simulink model "ES229A_HwTqCorrln"  (R2013b)
settings: Solver=FixedStepDiscrete  SolverMode=SingleTasking  StartTime=0.0  StopTime=1  FixedStep=0.002  RelTol=1e-3
undefined symbols (not defined in the file): ARCHGLBPRM_100MILLISEC_SEC_F32, FLTINJ_HWTQCORRLN_HWTQIDPTSIG, HwTqCorrlnChACmnModCmpLpFilActvnThd, HwTqCorrlnChACmnModCmpLpFilOutpLim, HwTqCorrlnChAImdtCorrlnChkFailThd, HwTqCorrlnChAImdtCorrlnChkPassThd, HwTqCorrlnChAStabStClrFltThd, HwTqCorrlnChAStabStSetFltThd, HwTqCorrlnChATqSumMaxLim, HwTqCorrlnChATraSumClrFltThd, HwTqCorrlnChATraSumSetFltThd, HwTqCorrlnChBCmnModCmpLpFilActvnThd, HwTqCorrlnChBCmnModCmpLpFilOutpLim, HwTqCorrlnChBImdtCorrlnChkFailThd, HwTqCorrlnChBImdtCorrlnChkPassThd, HwTqCorrlnChBStabStClrFltThd, HwTqCorrlnChBStabStSetFltThd, HwTqCorrlnChBTqSumMaxLim, HwTqCorrlnChBTraSumClrFltThd, HwTqCorrlnChBTraSumSetFltThd, HwTqCorrlnMaxStallTqA, HwTqCorrlnMaxStallTqB, HwTqCorrlnMaxStallTqC, HwTqCorrlnMaxStallTqD, HWTQSCA_CNT_U08, NtcNr1, NtcSts1, PARAMETERBYTE_CNT_U08, sigbuilder_block, SigQlfr1, STABSTLPFILSTVARIDELTALIM_HWNWTMTR_F32
libraries: simulink x25, Fil x12, NxtrLim x10, NxtrAbslt x6, FixdToFloat x2, FloatToFixdWithRound x2, LnrIntrpn x2, NxtrNvM x2
(part 3 of 4)

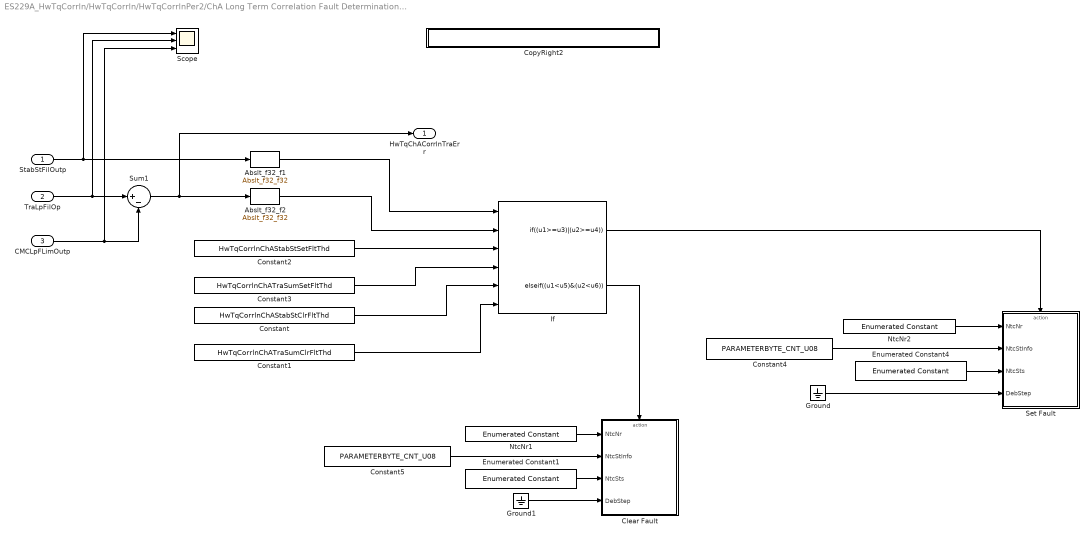
== system ES229A_HwTqCorrln/HwTqCorrln/HwTqCorrlnPer2/ChA Long Term Correlation Fault Determination/Ch A Set//Clear Fault ==
  StabStFilOutp : Inport
  TraLpFilOp : Inport  Port=2
  CMCLpFLimOutp : Inport  Port=3
  Abslt_f32_f1 : NxtrAbslt/Abslt_f32_f32  SFunctionSpec=single y1 = Abslt_f32_f32(single u1)
      settings: AttributesFormatString=%<Name>
  Abslt_f32_f2 : NxtrAbslt/Abslt_f32_f32  SFunctionSpec=single y1 = Abslt_f32_f32(single u1)
      settings: AttributesFormatString=%<Name>
  Clear Fault : Subsystem  mask(SetNTC){}
      mask help: SetNTC library block
  Constant : Constant  Value=HwTqCorrlnChAStabStClrFltThd
  Constant1 : Constant  Value=HwTqCorrlnChATraSumClrFltThd
  Constant2 : Constant  Value=HwTqCorrlnChAStabStSetFltThd
  Constant3 : Constant  Value=HwTqCorrlnChATraSumSetFltThd
  Constant4 : Constant  Value=PARAMETERBYTE_CNT_U08
  Constant5 : Constant  Value=PARAMETERBYTE_CNT_U08
  CopyRight2 : Subsystem  Description=|  mask(Copyright Information){none=on}
      | Copyright info block.                                               
      |                                                                     
      | Place copyright information at the top of every subsystem in design.
      mask prompts: none "No parameters"
      mask help: Place copyright information at the top of every subsystem in design.
      mask Display:
      | NxtrConf = 'Nexteer Confidential';
      | 
      | sys = bdroot; %handle for the current model ("system")
      | first = get_param(sys,'Created');
      | first = first(end-3:end);  %year is last four digits
      | 
      | last = get_param(sys,'LastModifiedDate');
      | if isempty(last)
      |     last = datestr(now,'yyyy');
      | else
      |     last = last(end-3:end);
      | end
      | 
      | if strcmp(first,last)
      |     fprintf('%s -- Copyright %s Nexteer',NxtrConf,first)
      | else
      |     fprintf('%s -- %s%s- %s Nexteer',NxtrConf,char(169),first,last)
      | end
  Enumerated Constant1 : simulink/Sources/Enumerated Constant  OutDataTypeStr=Enum: NtcSts1  Value=NtcSts1.NTCSTS_PASSD  SampleTime=inf
  Enumerated Constant4 : simulink/Sources/Enumerated Constant  OutDataTypeStr=Enum: NtcSts1  Value=NtcSts1.NTCSTS_FAILD  SampleTime=inf
  Ground : Ground
  Ground1 : Ground
  If : If  NumInputs=6  IfExpression=(u1>=u3)|(u2>=u4)  ElseIfExpressions=(u1<u5)&(u2<u6)  ShowElse=off
  NtcNr1 : simulink/Sources/Enumerated Constant  OutDataTypeStr=Enum: NtcNr1  Value=NtcNr1.NTCNR_0X070  SampleTime=inf
  NtcNr2 : simulink/Sources/Enumerated Constant  OutDataTypeStr=Enum: NtcNr1  Value=NtcNr1.NTCNR_0X070  SampleTime=inf
  Scope : Scope  NumInputPorts=3
      settings: TimeRange=auto  LimitDataPoints=on  MaxDataPoints=5000  SaveToWorkspace=off  SaveName=ScopeData3  YMin=-5~-5~-5  YMax=5~5~5  SampleTime=-1
  Set Fault : Subsystem  mask(SetNTC){}
      mask help: SetNTC library block
  Sum1 : Sum  RequirementInfo={} %GIDa_36dd93a3_b811_40f0_b925_6a2a9cd5f46c  Inputs=|+-
  HwTqChACorrlnTraErr : Outport
  wires:
  Abslt_f32_f1/1 -> If/1
  Constant/1 -> If/5
  Constant1/1 -> If/6
  If/1 -> Set Fault/Action
  NtcNr2/1 -> Set Fault/1(NtcNr)
  Constant4/1 -> Set Fault/2(NtcStInfo)
  Enumerated Constant4/1 -> Set Fault/3(NtcSts)
  Ground/1 -> Set Fault/4(DebStep)
  Constant3/1 -> If/4
  If/2 -> Clear Fault/Action
  NtcNr1/1 -> Clear Fault/1(NtcNr)
  Constant5/1 -> Clear Fault/2(NtcStInfo)
  Enumerated Constant1/1 -> Clear Fault/3(NtcSts)
  Ground1/1 -> Clear Fault/4(DebStep)
  StabStFilOutp/1 -> Scope/1, Abslt_f32_f1/1
  Sum1/1 -> HwTqChACorrlnTraErr/1, Abslt_f32_f2/1
  Abslt_f32_f2/1 -> If/2
  Constant2/1 -> If/3
  CMCLpFLimOutp/1 -> Scope/3, Sum1/2
  TraLpFilOp/1 -> Scope/2, Sum1/1

== system ES229A_HwTqCorrln/HwTqCorrln/HwTqCorrlnPer2/ChA Long Term Correlation Fault Determination/Ch A Variable Fc Transient Fault LPF ==
  note: Add data type conversion Inp and out of table
  TrqSumLmt : Inport
  Abslt_f32_f32 : NxtrAbslt/Abslt_f32_f32  SFunctionSpec=single y1 = Abslt_f32_f32(single u1)
      settings: AttributesFormatString=%<Name>
  CopyRight2 : Subsystem  Description=|  mask(Copyright Information){none=on}
      | Copyright info block.                                               
      |                                                                     
      | Place copyright information at the top of every subsystem in design.
      mask prompts: none "No parameters"
      mask help: Place copyright information at the top of every subsystem in design.
      mask Display:
      | NxtrConf = 'Nexteer Confidential';
      | 
      | sys = bdroot; %handle for the current model ("system")
      | first = get_param(sys,'Created');
      | first = first(end-3:end);  %year is last four digits
      | 
      | last = get_param(sys,'LastModifiedDate');
      | if isempty(last)
      |     last = datestr(now,'yyyy');
      | else
      |     last = last(end-3:end);
      | end
      | 
      | if strcmp(first,last)
      |     fprintf('%s -- Copyright %s Nexteer',NxtrConf,first)
      | else
      |     fprintf('%s -- %s%s- %s Nexteer',NxtrConf,char(169),first,last)
      | end
  FilLpUpdGain : Fil/FilLpUpdGain  Priority=2  Ts=single(0.004)  StVar=HwTqChATraLpFil
      settings: AttributesFormatString=|
      | Ts: %<Ts>
      | StVar: %<StVar>
      | Priority: %<Priority>
  FilLpUpdOutp : Fil/FilLpUpdOutp  Priority=3  StVar=HwTqChATraLpFil
      settings: AttributesFormatString=|
      | StVar: %<StVar>
      | Priority: %<Priority>
  FixdToFloat_f32_u16 : FixdToFloat/FixdToFloat_f32_u16  Param1=10
  FloatToFixdWithRound_u16_f32 : FloatToFixdWithRound/FloatToFixdWithRound_u16_f32  Param1=11
  LnrIntrpn_u16_u16VariXu16VariY : LnrIntrpn/LnrIntrpn_u16_u16VariXu16VariY  Priority=1  XTbl=HwTqCorrlnChATraLpFilX  YTbl=HwTqCorrlnChATraLpFilY
      settings: AttributesFormatString=|
      | Lnr ( u16VariX , u16VariY )
      | Priority: %<Priority>
  TraLpFilOp : Outport
  wires:
  TrqSumLmt/1 -> Abslt_f32_f32/1, FilLpUpdOutp/1
  Abslt_f32_f32/1 -> FloatToFixdWithRound_u16_f32/1
  LnrIntrpn_u16_u16VariXu16VariY/1 -> FixdToFloat_f32_u16/1
  FloatToFixdWithRound_u16_f32/1 -> LnrIntrpn_u16_u16VariXu16VariY/1
  FixdToFloat_f32_u16/1 -> FilLpUpdGain/1
  FilLpUpdOutp/1 -> TraLpFilOp/1

== system ES229A_HwTqCorrln/HwTqCorrln/HwTqCorrlnPer2/ChA Long Term Correlation Fault Determination/ChA CMC LPF Limit ==
  Constant1 : Constant  RequirementInfo={} %GIDa_72eaf94a_e667_4cbf_a56b_a3f43667705d  Value=-1  OutDataTypeStr=single
  Constant2 : Constant  RequirementInfo={} %GIDa_dca1123b_deb2_4786_b31b_bd2c5c60cbec  Value=HwTqCorrlnChACmnModCmpLpFilOutpLim
  CopyRight2 : Subsystem  Description=|  mask(Copyright Information){none=on}
      | Copyright info block.                                               
      |                                                                     
      | Place copyright information at the top of every subsystem in design.
      mask prompts: none "No parameters"
      mask help: Place copyright information at the top of every subsystem in design.
      mask Display:
      | NxtrConf = 'Nexteer Confidential';
      | 
      | sys = bdroot; %handle for the current model ("system")
      | first = get_param(sys,'Created');
      | first = first(end-3:end);  %year is last four digits
      | 
      | last = get_param(sys,'LastModifiedDate');
      | if isempty(last)
      |     last = datestr(now,'yyyy');
      | else
      |     last = last(end-3:end);
      | end
      | 
      | if strcmp(first,last)
      |     fprintf('%s -- Copyright %s Nexteer',NxtrConf,first)
      | else
      |     fprintf('%s -- %s%s- %s Nexteer',NxtrConf,char(169),first,last)
      | end
  Data Store Read1 : DataStoreRead  DataStoreName=HwTqChACmnModCmpLpFil  DataStoreElements=HwTqChACmnModCmpLpFil.FilSt
  LimDyn_f32 : NxtrLim/LimDyn_f32  RequirementInfo={} %GIDa_1c7be57d_faef_4bd1_a7ab_75ed3e2b2752
  Product : Product  RequirementInfo={} %GIDa_d7a373ed_dd9b_4899_a765_22120a24fae2  OutDataTypeStr=single
  CmnModCmpLpFilOutpLmt : Outport
  wires:
  LimDyn_f32/1 -> CmnModCmpLpFilOutpLmt/1
  Data Store Read1/1 -> LimDyn_f32/1
  Constant2/1 -> Product/2, LimDyn_f32/3
  Constant1/1 -> Product/1
  Product/1 -> LimDyn_f32/2

== system ES229A_HwTqCorrln/HwTqCorrln/HwTqCorrlnPer2/ChA Long Term Correlation Fault Determination/ChA Trq Sum Limit ==
  In1 : Inport
  In2 : Inport  Port=2
  Constant : Constant  Value=HWTQSCA_CNT_U08
  Constant1 : Constant  Value=-1  OutDataTypeStr=single
  Constant3 : Constant  RequirementInfo={} %GIDa_078b91aa_a9cb_4a51_ac3c_bc7f46b72b6a  Value=HwTqCorrlnChATqSumMaxLim
  CopyRight2 : Subsystem  Description=|  mask(Copyright Information){none=on}
      | Copyright info block.                                               
      |                                                                     
      | Place copyright information at the top of every subsystem in design.
      mask prompts: none "No parameters"
      mask help: Place copyright information at the top of every subsystem in design.
      mask Display:
      | NxtrConf = 'Nexteer Confidential';
      | 
      | sys = bdroot; %handle for the current model ("system")
      | first = get_param(sys,'Created');
      | first = first(end-3:end);  %year is last four digits
      | 
      | last = get_param(sys,'LastModifiedDate');
      | if isempty(last)
      |     last = datestr(now,'yyyy');
      | else
      |     last = last(end-3:end);
      | end
      | 
      | if strcmp(first,last)
      |     fprintf('%s -- Copyright %s Nexteer',NxtrConf,first)
      | else
      |     fprintf('%s -- %s%s- %s Nexteer',NxtrConf,char(169),first,last)
      | end
  Divide : Product  Inputs=*/
  LimDyn_f32 : NxtrLim/LimDyn_f32
  Product : Product  OutDataTypeStr=single
  Sum : Sum  Inputs=+|-
  Out1 : Outport
  wires:
  In1/1 -> Sum/1
  In2/1 -> Sum/2
  Sum/1 -> Divide/1
  Divide/1 -> LimDyn_f32/1  "TrqSum"
  Constant/1 -> Divide/2
  Constant1/1 -> Product/1
  Product/1 -> LimDyn_f32/2
  LimDyn_f32/1 -> Out1/1
  Constant3/1 -> Product/2, LimDyn_f32/3

== system ES229A_HwTqCorrln/HwTqCorrln/HwTqCorrlnPer2/ChA Long Term Correlation Fault Determination/CopyRight2 ==

== system ES229A_HwTqCorrln/HwTqCorrln/HwTqCorrlnPer2/ChB Long Term Correlation Fault Determination/Ch B CMC LPF Limit ==
  Constant1 : Constant  RequirementInfo={} %GIDa_4157bb2a_3465_479c_bcd4_5c172c793f58  Value=-1  OutDataTypeStr=single
  Constant2 : Constant  RequirementInfo={} %GIDa_3cadad4c_0ad0_4f07_8e93_f8e6371f4d2e  Value=HwTqCorrlnChBCmnModCmpLpFilOutpLim
  CopyRight2 : Subsystem  Description=|  mask(Copyright Information){none=on}
      | Copyright info block.                                               
      |                                                                     
      | Place copyright information at the top of every subsystem in design.
      mask prompts: none "No parameters"
      mask help: Place copyright information at the top of every subsystem in design.
      mask Display:
      | NxtrConf = 'Nexteer Confidential';
      | 
      | sys = bdroot; %handle for the current model ("system")
      | first = get_param(sys,'Created');
      | first = first(end-3:end);  %year is last four digits
      | 
      | last = get_param(sys,'LastModifiedDate');
      | if isempty(last)
      |     last = datestr(now,'yyyy');
      | else
      |     last = last(end-3:end);
      | end
      | 
      | if strcmp(first,last)
      |     fprintf('%s -- Copyright %s Nexteer',NxtrConf,first)
      | else
      |     fprintf('%s -- %s%s- %s Nexteer',NxtrConf,char(169),first,last)
      | end
  Data Store Read1 : DataStoreRead  DataStoreName=HwTqChBCmnModCmpLpFil  DataStoreElements=HwTqChBCmnModCmpLpFil.FilSt
  LimDyn_f32 : NxtrLim/LimDyn_f32  RequirementInfo={} %GIDa_b7b007e8_1625_44f1_bce4_ff77f2350629
  Product : Product  RequirementInfo={} %GIDa_cff75b14_a24a_481f_8bd3_5d42033c7938
  CmnModCmpLpFilOutpLmt : Outport
  wires:
  LimDyn_f32/1 -> CmnModCmpLpFilOutpLmt/1
  Data Store Read1/1 -> LimDyn_f32/1
  Constant2/1 -> Product/2, LimDyn_f32/3
  Constant1/1 -> Product/1
  Product/1 -> LimDyn_f32/2

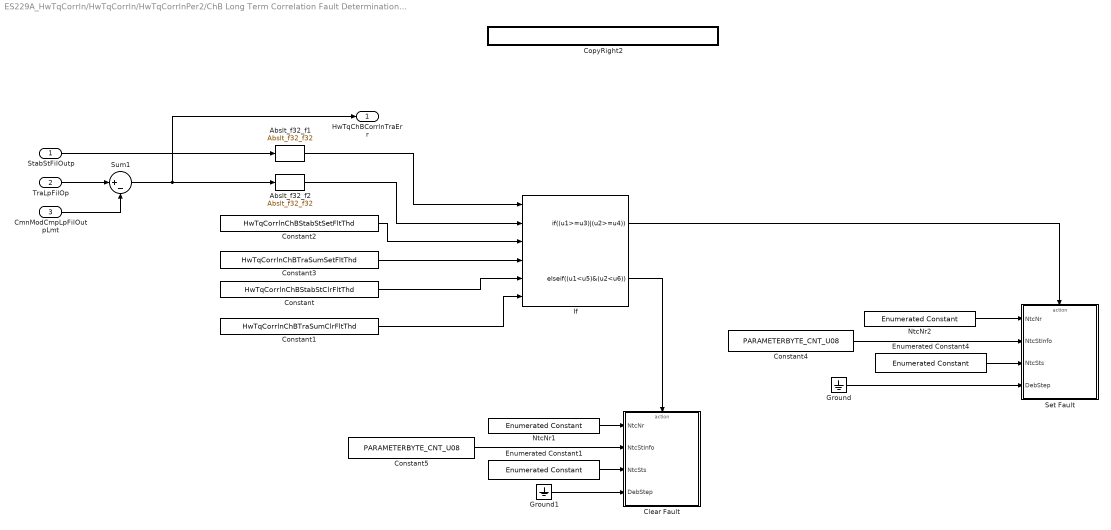
== system ES229A_HwTqCorrln/HwTqCorrln/HwTqCorrlnPer2/ChB Long Term Correlation Fault Determination/Ch B Set//Clear Fault ==
  StabStFilOutp : Inport
  TraLpFilOp : Inport  Port=2
  CmnModCmpLpFilOutpLmt : Inport  Port=3
  Abslt_f32_f1 : NxtrAbslt/Abslt_f32_f32  SFunctionSpec=single y1 = Abslt_f32_f32(single u1)
      settings: AttributesFormatString=%<Name>
  Abslt_f32_f2 : NxtrAbslt/Abslt_f32_f32  SFunctionSpec=single y1 = Abslt_f32_f32(single u1)
      settings: AttributesFormatString=%<Name>
  Clear Fault : Subsystem  mask(SetNTC){}
      mask help: SetNTC library block
  Constant : Constant  Value=HwTqCorrlnChBStabStClrFltThd
  Constant1 : Constant  Value=HwTqCorrlnChBTraSumClrFltThd
  Constant2 : Constant  Value=HwTqCorrlnChBStabStSetFltThd
  Constant3 : Constant  Value=HwTqCorrlnChBTraSumSetFltThd
  Constant4 : Constant  Value=PARAMETERBYTE_CNT_U08
  Constant5 : Constant  Value=PARAMETERBYTE_CNT_U08
  CopyRight2 : Subsystem  Description=|  mask(Copyright Information){none=on}
      | Copyright info block.                                               
      |                                                                     
      | Place copyright information at the top of every subsystem in design.
      mask prompts: none "No parameters"
      mask help: Place copyright information at the top of every subsystem in design.
      mask Display:
      | NxtrConf = 'Nexteer Confidential';
      | 
      | sys = bdroot; %handle for the current model ("system")
      | first = get_param(sys,'Created');
      | first = first(end-3:end);  %year is last four digits
      | 
      | last = get_param(sys,'LastModifiedDate');
      | if isempty(last)
      |     last = datestr(now,'yyyy');
      | else
      |     last = last(end-3:end);
      | end
      | 
      | if strcmp(first,last)
      |     fprintf('%s -- Copyright %s Nexteer',NxtrConf,first)
      | else
      |     fprintf('%s -- %s%s- %s Nexteer',NxtrConf,char(169),first,last)
      | end
  Enumerated Constant1 : simulink/Sources/Enumerated Constant  OutDataTypeStr=Enum: NtcSts1  Value=NtcSts1.NTCSTS_PASSD  SampleTime=inf
  Enumerated Constant4 : simulink/Sources/Enumerated Constant  OutDataTypeStr=Enum: NtcSts1  Value=NtcSts1.NTCSTS_FAILD  SampleTime=inf
  Ground : Ground
  Ground1 : Ground
  If : If  NumInputs=6  IfExpression=(u1>=u3)|(u2>=u4)  ElseIfExpressions=(u1<u5)&(u2<u6)  ShowElse=off
  NtcNr1 : simulink/Sources/Enumerated Constant  OutDataTypeStr=Enum: NtcNr1  Value=NtcNr1.NTCNR_0X071  SampleTime=inf
  NtcNr2 : simulink/Sources/Enumerated Constant  OutDataTypeStr=Enum: NtcNr1  Value=NtcNr1.NTCNR_0X071  SampleTime=inf
  Set Fault : Subsystem  mask(SetNTC){}
      mask help: SetNTC library block
  Sum1 : Sum  RequirementInfo={} %GIDa_fee84713_1c6a_4cf6_b4c8_2687f636226d  Inputs=|+-
  HwTqChBCorrlnTraErr : Outport
  wires:
  Abslt_f32_f1/1 -> If/1
  Constant/1 -> If/5
  Constant1/1 -> If/6
  If/1 -> Set Fault/Action
  NtcNr2/1 -> Set Fault/1(NtcNr)
  Constant4/1 -> Set Fault/2(NtcStInfo)
  Enumerated Constant4/1 -> Set Fault/3(NtcSts)
  Ground/1 -> Set Fault/4(DebStep)
  Constant3/1 -> If/4
  If/2 -> Clear Fault/Action
  NtcNr1/1 -> Clear Fault/1(NtcNr)
  Constant5/1 -> Clear Fault/2(NtcStInfo)
  Enumerated Constant1/1 -> Clear Fault/3(NtcSts)
  Ground1/1 -> Clear Fault/4(DebStep)
  StabStFilOutp/1 -> Abslt_f32_f1/1
  TraLpFilOp/1 -> Sum1/1
  Abslt_f32_f2/1 -> If/2
  Constant2/1 -> If/3
  CmnModCmpLpFilOutpLmt/1 -> Sum1/2
  Sum1/1 -> HwTqChBCorrlnTraErr/1, Abslt_f32_f2/1

== system ES229A_HwTqCorrln/HwTqCorrln/HwTqCorrlnPer2/ChB Long Term Correlation Fault Determination/Ch B Variable Fc Transient Fault LPF ==
  TrqSumLmt : Inport
  Abslt_f32_f32 : NxtrAbslt/Abslt_f32_f32  SFunctionSpec=single y1 = Abslt_f32_f32(single u1)
      settings: AttributesFormatString=%<Name>
  CopyRight2 : Subsystem  Description=|  mask(Copyright Information){none=on}
      | Copyright info block.                                               
      |                                                                     
      | Place copyright information at the top of every subsystem in design.
      mask prompts: none "No parameters"
      mask help: Place copyright information at the top of every subsystem in design.
      mask Display:
      | NxtrConf = 'Nexteer Confidential';
      | 
      | sys = bdroot; %handle for the current model ("system")
      | first = get_param(sys,'Created');
      | first = first(end-3:end);  %year is last four digits
      | 
      | last = get_param(sys,'LastModifiedDate');
      | if isempty(last)
      |     last = datestr(now,'yyyy');
      | else
      |     last = last(end-3:end);
      | end
      | 
      | if strcmp(first,last)
      |     fprintf('%s -- Copyright %s Nexteer',NxtrConf,first)
      | else
      |     fprintf('%s -- %s%s- %s Nexteer',NxtrConf,char(169),first,last)
      | end
  FilLpUpdGain : Fil/FilLpUpdGain  Priority=2  Ts=single(0.004)  StVar=HwTqChBTraLpFil
      settings: AttributesFormatString=|
      | Ts: %<Ts>
      | StVar: %<StVar>
      | Priority: %<Priority>
  FilLpUpdOutp : Fil/FilLpUpdOutp  Priority=3  StVar=HwTqChBTraLpFil
      settings: AttributesFormatString=|
      | StVar: %<StVar>
      | Priority: %<Priority>
  FixdToFloat_f32_u16 : FixdToFloat/FixdToFloat_f32_u16  Param1=10
  FloatToFixdWithRound_u16_f32 : FloatToFixdWithRound/FloatToFixdWithRound_u16_f32  Param1=11
  LnrIntrpn_u16_u16VariXu16VariY : LnrIntrpn/LnrIntrpn_u16_u16VariXu16VariY  Priority=1  XTbl=HwTqCorrlnChBTraLpFilX  YTbl=HwTqCorrlnChBTraLpFilY
      settings: AttributesFormatString=|
      | Lnr ( u16VariX , u16VariY )
      | Priority: %<Priority>
  TraLpFilOp : Outport
  wires:
  TrqSumLmt/1 -> FilLpUpdOutp/1, Abslt_f32_f32/1
  FloatToFixdWithRound_u16_f32/1 -> LnrIntrpn_u16_u16VariXu16VariY/1
  LnrIntrpn_u16_u16VariXu16VariY/1 -> FixdToFloat_f32_u16/1
  FilLpUpdOutp/1 -> TraLpFilOp/1
  Abslt_f32_f32/1 -> FloatToFixdWithRound_u16_f32/1
  FixdToFloat_f32_u16/1 -> FilLpUpdGain/1

== system ES229A_HwTqCorrln/HwTqCorrln/HwTqCorrlnPer2/ChB Long Term Correlation Fault Determination/ChB Trq Sum Limit ==
  In1 : Inport
  In2 : Inport  Port=2
  Constant : Constant  Value=HWTQSCA_CNT_U08
  Constant1 : Constant  Value=-1  OutDataTypeStr=single
  Constant3 : Constant  RequirementInfo={} %GIDa_d58f60e6_8b98_4825_9fd0_1ecc30478779  Value=HwTqCorrlnChBTqSumMaxLim
  CopyRight2 : Subsystem  Description=|  mask(Copyright Information){none=on}
      | Copyright info block.                                               
      |                                                                     
      | Place copyright information at the top of every subsystem in design.
      mask prompts: none "No parameters"
      mask help: Place copyright information at the top of every subsystem in design.
      mask Display:
      | NxtrConf = 'Nexteer Confidential';
      | 
      | sys = bdroot; %handle for the current model ("system")
      | first = get_param(sys,'Created');
      | first = first(end-3:end);  %year is last four digits
      | 
      | last = get_param(sys,'LastModifiedDate');
      | if isempty(last)
      |     last = datestr(now,'yyyy');
      | else
      |     last = last(end-3:end);
      | end
      | 
      | if strcmp(first,last)
      |     fprintf('%s -- Copyright %s Nexteer',NxtrConf,first)
      | else
      |     fprintf('%s -- %s%s- %s Nexteer',NxtrConf,char(169),first,last)
      | end
  Divide : Product  Inputs=*/
  LimDyn_f32 : NxtrLim/LimDyn_f32
  Product : Product  OutDataTypeStr=single
  Sum : Sum  Inputs=+|-
  Out1 : Outport
  wires:
  In1/1 -> Sum/1
  In2/1 -> Sum/2
  Sum/1 -> Divide/1
  Divide/1 -> LimDyn_f32/1  "TrqSum"
  Constant/1 -> Divide/2
  Constant1/1 -> Product/1
  Product/1 -> LimDyn_f32/2
  LimDyn_f32/1 -> Out1/1
  Constant3/1 -> Product/2, LimDyn_f32/3

== system ES229A_HwTqCorrln/HwTqCorrln/HwTqCorrlnPer2/ChB Long Term Correlation Fault Determination/CopyRight2 ==

== system ES229A_HwTqCorrln/HwTqCorrln/HwTqCorrlnPer2/Independent Signals Determination/CopyRight2 ==

== system ES229A_HwTqCorrln/HwTqCorrln/HwTqCorrlnPer2/Independent Signals Determination/GetNtcQlfrSts ==
  NtcNr : Inport
  CopyRight2 : Subsystem  Description=|  mask(Copyright Information){none=on}
      | Copyright info block.                                               
      |                                                                     
      | Place copyright information at the top of every subsystem in design.
      mask prompts: none "No parameters"
      mask help: Place copyright information at the top of every subsystem in design.
      mask Display:
      | NxtrConf = 'Nexteer Confidential';
      | 
      | sys = bdroot; %handle for the current model ("system")
      | first = get_param(sys,'Created');
      | first = first(end-3:end);  %year is last four digits
      | 
      | last = get_param(sys,'LastModifiedDate');
      | if isempty(last)
      |     last = datestr(now,'yyyy');
      | else
      |     last = last(end-3:end);
      | end
      | 
      | if strcmp(first,last)
      |     fprintf('%s -- Copyright %s Nexteer',NxtrConf,first)
      | else
      |     fprintf('%s -- %s%s- %s Nexteer',NxtrConf,char(169),first,last)
      | end
  Data Store Read : DataStoreRead  DataStoreName=NtcQlfr0x70
  Terminator : Terminator
  NtcQlfr : Outport
  wires:
  NtcNr/1 -> Terminator/1
  Data Store Read/1 -> NtcQlfr/1

== system ES229A_HwTqCorrln/HwTqCorrln/HwTqCorrlnPer2/Independent Signals Determination/GetNtcQlfrSts1 ==
  NtcNr : Inport
  CopyRight2 : Subsystem  Description=|  mask(Copyright Information){none=on}
      | Copyright info block.                                               
      |                                                                     
      | Place copyright information at the top of every subsystem in design.
      mask prompts: none "No parameters"
      mask help: Place copyright information at the top of every subsystem in design.
      mask Display:
      | NxtrConf = 'Nexteer Confidential';
      | 
      | sys = bdroot; %handle for the current model ("system")
      | first = get_param(sys,'Created');
      | first = first(end-3:end);  %year is last four digits
      | 
      | last = get_param(sys,'LastModifiedDate');
      | if isempty(last)
      |     last = datestr(now,'yyyy');
      | else
      |     last = last(end-3:end);
      | end
      | 
      | if strcmp(first,last)
      |     fprintf('%s -- Copyright %s Nexteer',NxtrConf,first)
      | else
      |     fprintf('%s -- %s%s- %s Nexteer',NxtrConf,char(169),first,last)
      | end
  Data Store Read : DataStoreRead  DataStoreName=NtcQlfr
  Terminator : Terminator
  NtcQlfr : Outport
  wires:
  NtcNr/1 -> Terminator/1
  Data Store Read/1 -> NtcQlfr/1

== system ES229A_HwTqCorrln/HwTqCorrln/HwTqCorrlnPer3/ChA Long Term Offset Compensation/ChA CMC LPF ==
  In1 : Inport
  TqSumLmt : Inport  RequirementInfo={} %GIDa_fbcd160a_d5f0_4e4e_b1ee_e3a574d62016  Port=2
  Abs1 : Abs  RequirementInfo={} %GIDa_8c8f43dc_2cf0_4714_8275_f28598b547f6
  Ch A CMC LPF Hold Last Val : Subsystem  RequirementInfo={} %GIDa_01f2f491_961f_41b5_9cb7_8045637af8b5  TreatAsAtomicUnit=on
  Ch A CMC LPF Update Outp : Subsystem  RequirementInfo={} %GIDa_1d19e8fd_8a20_477c_96b5_c46bfeecd0f1  TreatAsAtomicUnit=on
  Constant1 : Constant
  Constant2 : Constant  RequirementInfo={} %GIDa_49ab2ba3_1f9c_4ed3_89f8_1ba8a00fbf62  Value=HwTqCorrlnChACmnModCmpLpFilActvnThd
  CopyRight2 : Subsystem  Description=|  mask(Copyright Information){none=on}
      | Copyright info block.                                               
      |                                                                     
      | Place copyright information at the top of every subsystem in design.
      mask prompts: none "No parameters"
      mask help: Place copyright information at the top of every subsystem in design.
      mask Display:
      | NxtrConf = 'Nexteer Confidential';
      | 
      | sys = bdroot; %handle for the current model ("system")
      | first = get_param(sys,'Created');
      | first = first(end-3:end);  %year is last four digits
      | 
      | last = get_param(sys,'LastModifiedDate');
      | if isempty(last)
      |     last = datestr(now,'yyyy');
      | else
      |     last = last(end-3:end);
      | end
      | 
      | if strcmp(first,last)
      |     fprintf('%s -- Copyright %s Nexteer',NxtrConf,first)
      | else
      |     fprintf('%s -- %s%s- %s Nexteer',NxtrConf,char(169),first,last)
      | end
  Data Store Write NVM Shadowed RAM : DataStoreWrite  RequirementInfo="{'linktype_rmi_doors' '0000c477 (/ESG Group/FDD Module Requirements/EA4 Specific/ES229A_HwTqCorrln)' '#ES229A_108' 'true' 'REQ:  ES229A_108' '' } %GIDa_4068a6b9_91f5_416d_8d33_1d0921b48612"  DataStoreName=HwTqChACmnModCmpLpFilSt
  If : If  RequirementInfo={} %GIDa_218a0e38_50f6_4f23_b972_fe92a00e6aad  IfExpression=u1==1
  Merge : Merge
  Relational Operator : RelationalOperator  RequirementInfo={} %GIDa_381ed7a9_b483_4eb6_bf4b_a3b90f176eaa  Operator=<  OutDataTypeStr=boolean
  Set Ram Block Status : NxtrNvM/Set Ram Block Status  RequirementInfo="{'linktype_rmi_doors' '0000c477 (/ESG Group/FDD Module Requirements/EA4 Specific/ES229A_HwTqCorrln)' '#ES229A_108' 'true' 'REQ:  ES229A_108' '' } %GIDa_247c9a98_4d53_4593_b5f6_0ba49b9ca8e1"  FuncName=Set Ram Block Status  NvMBlockName=HwTqChACmnModCmpLpFilSt  VoidFuncRtn=on  BlockChanged_DSN=NvMSRBS_BlockChanged  Return_DSN=NvMSRBS_Return
      settings: AttributesFormatString=%<FuncName>
  wires:
  In1/1 -> Abs1/1
  Abs1/1 -> Relational Operator/1
  Constant2/1 -> Relational Operator/2
  Relational Operator/1 -> If/1
  TqSumLmt/1 -> Ch A CMC LPF Update Outp/1(In1)
  If/1 -> Ch A CMC LPF Update Outp/Action
  Merge/1 -> Data Store Write NVM Shadowed RAM/1
  Ch A CMC LPF Update Outp/1(Out1) -> Merge/1
  Ch A CMC LPF Hold Last Val/1(Out1) -> Merge/2
  If/2 -> Ch A CMC LPF Hold Last Val/Action
  Constant1/1 -> Set Ram Block Status/1

== system ES229A_HwTqCorrln/HwTqCorrln/HwTqCorrlnPer3/ChA Long Term Offset Compensation/CopyRight1 ==

== system ES229A_HwTqCorrln/HwTqCorrln/HwTqCorrlnPer3/ChA Long Term Offset Compensation/CopyRight2 ==

== system ES229A_HwTqCorrln/HwTqCorrln/HwTqCorrlnPer3/ChA Long Term Offset Compensation/Limit StabStLPF Output ==
  In1 : Inport
  Constant : Constant  Value=HwTqCorrlnChAStabStSetFltThd
  Constant1 : Constant  Value=STABSTLPFILSTVARIDELTALIM_HWNWTMTR_F32
  Constant2 : Constant  Value=-1  OutDataTypeStr=single
  CopyRight2 : Subsystem  Description=|  mask(Copyright Information){none=on}
      | Copyright info block.                                               
      |                                                                     
      | Place copyright information at the top of every subsystem in design.
      mask prompts: none "No parameters"
      mask help: Place copyright information at the top of every subsystem in design.
      mask Display:
      | NxtrConf = 'Nexteer Confidential';
      | 
      | sys = bdroot; %handle for the current model ("system")
      | first = get_param(sys,'Created');
      | first = first(end-3:end);  %year is last four digits
      | 
      | last = get_param(sys,'LastModifiedDate');
      | if isempty(last)
      |     last = datestr(now,'yyyy');
      | else
      |     last = last(end-3:end);
      | end
      | 
      | if strcmp(first,last)
      |     fprintf('%s -- Copyright %s Nexteer',NxtrConf,first)
      | else
      |     fprintf('%s -- %s%s- %s Nexteer',NxtrConf,char(169),first,last)
      | end
  LimDyn_f32 : NxtrLim/LimDyn_f32
  Product : Product
  Sum : Sum  Inputs=|++
  Out1 : Outport
  wires:
  In1/1 -> LimDyn_f32/1
  Constant/1 -> Sum/1
  Constant1/1 -> Sum/2
  Sum/1 -> LimDyn_f32/3, Product/2
  Constant2/1 -> Product/1
  Product/1 -> LimDyn_f32/2
  LimDyn_f32/1 -> Out1/1

== system ES229A_HwTqCorrln/HwTqCorrln/HwTqCorrlnPer3/ChB Long Term Offset Compensation/ChB CMC LPF ==
  In1 : Inport
  In2 : Inport  Port=2
  Abs1 : Abs  RequirementInfo={} %GIDa_c1d07f50_2202_4831_a53f_b93704718eb6
  Ch B CMC LPF Hold Last Val : Subsystem  RequirementInfo={} %GIDa_97de0faf_7c71_4616_b041_fc7d37ab5f2b  TreatAsAtomicUnit=on
  Ch B CMC LPF Update Outp : Subsystem  RequirementInfo={} %GIDa_9ceae595_2085_4f0b_b0f0_3f68cec57c15  TreatAsAtomicUnit=on
  Constant1 : Constant
  Constant2 : Constant  RequirementInfo={} %GIDa_e94b1530_8388_4048_a94c_adf2bc40370e  Value=HwTqCorrlnChBCmnModCmpLpFilActvnThd
  CopyRight2 : Subsystem  Description=|  mask(Copyright Information){none=on}
      | Copyright info block.                                               
      |                                                                     
      | Place copyright information at the top of every subsystem in design.
      mask prompts: none "No parameters"
      mask help: Place copyright information at the top of every subsystem in design.
      mask Display:
      | NxtrConf = 'Nexteer Confidential';
      | 
      | sys = bdroot; %handle for the current model ("system")
      | first = get_param(sys,'Created');
      | first = first(end-3:end);  %year is last four digits
      | 
      | last = get_param(sys,'LastModifiedDate');
      | if isempty(last)
      |     last = datestr(now,'yyyy');
      | else
      |     last = last(end-3:end);
      | end
      | 
      | if strcmp(first,last)
      |     fprintf('%s -- Copyright %s Nexteer',NxtrConf,first)
      | else
      |     fprintf('%s -- %s%s- %s Nexteer',NxtrConf,char(169),first,last)
      | end
  Data Store Write NVM Shadowed RAM : DataStoreWrite  RequirementInfo="{'linktype_rmi_doors' '0000c477 (/ESG Group/FDD Module Requirements/EA4 Specific/ES229A_HwTqCorrln)' '#ES229A_109' 'true' 'REQ:  ES229A_109' '' } %GIDa_be15f2d9_8e98_469c_994e_29fcb9382441"  DataStoreName=HwTqChBCmnModCmpLpFilSt
  If : If  RequirementInfo={} %GIDa_ae134f23_13cd_453f_bb39_22ab953eaf0b  IfExpression=u1==1
  Merge : Merge
  Relational Operator : RelationalOperator  RequirementInfo={} %GIDa_40ed6311_5ff1_443d_8439_2ddada0eb1de  Operator=<  OutDataTypeStr=boolean
  Set Ram Block Status : NxtrNvM/Set Ram Block Status  RequirementInfo="{'linktype_rmi_doors' '0000c477 (/ESG Group/FDD Module Requirements/EA4 Specific/ES229A_HwTqCorrln)' '#ES229A_109' 'true' 'REQ:  ES229A_109' '' } %GIDa_9caf7594_2e62_4d5e_a506_11c186b10ce5"  FuncName=Set Ram Block Status  NvMBlockName=HwTqChBCmnModCmpLpFilSt  VoidFuncRtn=on  BlockChanged_DSN=NvMSRBS_BlockChanged  Return_DSN=NvMSRBS_Return
      settings: AttributesFormatString=%<FuncName>
  wires:
  In1/1 -> Abs1/1
  Abs1/1 -> Relational Operator/1
  Constant2/1 -> Relational Operator/2
  Relational Operator/1 -> If/1
  In2/1 -> Ch B CMC LPF Update Outp/1(In1)
  If/1 -> Ch B CMC LPF Update Outp/Action
  Ch B CMC LPF Update Outp/1(Out1) -> Merge/1
  Ch B CMC LPF Hold Last Val/1(Out1) -> Merge/2
  If/2 -> Ch B CMC LPF Hold Last Val/Action
  Constant1/1 -> Set Ram Block Status/1
  Merge/1 -> Data Store Write NVM Shadowed RAM/1

== system ES229A_HwTqCorrln/HwTqCorrln/HwTqCorrlnPer3/ChB Long Term Offset Compensation/CopyRight2 ==

== system ES229A_HwTqCorrln/HwTqCorrln/HwTqCorrlnPer3/ChB Long Term Offset Compensation/Limit StabStLPF Output ==
  In1 : Inport
  Constant : Constant  Value=HwTqCorrlnChBStabStSetFltThd
  Constant1 : Constant  Value=STABSTLPFILSTVARIDELTALIM_HWNWTMTR_F32
  Constant2 : Constant  Value=-1  OutDataTypeStr=single
  CopyRight2 : Subsystem  Description=|  mask(Copyright Information){none=on}
      | Copyright info block.                                               
      |                                                                     
      | Place copyright information at the top of every subsystem in design.
      mask prompts: none "No parameters"
      mask help: Place copyright information at the top of every subsystem in design.
      mask Display:
      | NxtrConf = 'Nexteer Confidential';
      | 
      | sys = bdroot; %handle for the current model ("system")
      | first = get_param(sys,'Created');
      | first = first(end-3:end);  %year is last four digits
      | 
      | last = get_param(sys,'LastModifiedDate');
      | if isempty(last)
      |     last = datestr(now,'yyyy');
      | else
      |     last = last(end-3:end);
      | end
      | 
      | if strcmp(first,last)
      |     fprintf('%s -- Copyright %s Nexteer',NxtrConf,first)
      | else
      |     fprintf('%s -- %s%s- %s Nexteer',NxtrConf,char(169),first,last)
      | end
  LimDyn_f32 : NxtrLim/LimDyn_f32
  Product : Product
  Sum : Sum  Inputs=|++
  Out1 : Outport
  wires:
  In1/1 -> LimDyn_f32/1
  Constant/1 -> Sum/1
  Constant1/1 -> Sum/2
  Sum/1 -> LimDyn_f32/3, Product/2
  Constant2/1 -> Product/1
  Product/1 -> LimDyn_f32/2
  LimDyn_f32/1 -> Out1/1

== system ES229A_HwTqCorrln/HwTqCorrln/HwTqCorrlnPer1/ChA  Immediate Corrleation Check /Clear Corrln Bits/CopyRight2 ==

== system ES229A_HwTqCorrln/HwTqCorrln/HwTqCorrlnPer1/ChA  Immediate Corrleation Check /GetNtcQlfrSts/CopyRight2 ==

== system ES229A_HwTqCorrln/HwTqCorrln/HwTqCorrlnPer1/ChA  Immediate Corrleation Check /Set Corrln Bits/CopyRight2 ==

== system ES229A_HwTqCorrln/HwTqCorrln/HwTqCorrlnPer1/ChA  Immediate Corrleation Check /Signals Available/CopyRight2 ==

== system ES229A_HwTqCorrln/HwTqCorrln/HwTqCorrlnPer1/ChA  Immediate Corrleation Check /Signals Available/Hold last value ==
  Action Port : ActionPort  ActionType=else
  CopyRight2 : Subsystem  Description=|  mask(Copyright Information){none=on}
      | Copyright info block.                                               
      |                                                                     
      | Place copyright information at the top of every subsystem in design.
      mask prompts: none "No parameters"
      mask help: Place copyright information at the top of every subsystem in design.
      mask Display:
      | NxtrConf = 'Nexteer Confidential';
      | 
      | sys = bdroot; %handle for the current model ("system")
      | first = get_param(sys,'Created');
      | first = first(end-3:end);  %year is last four digits
      | 
      | last = get_param(sys,'LastModifiedDate');
      | if isempty(last)
      |     last = datestr(now,'yyyy');
      | else
      |     last = last(end-3:end);
      | end
      | 
      | if strcmp(first,last)
      |     fprintf('%s -- Copyright %s Nexteer',NxtrConf,first)
      | else
      |     fprintf('%s -- %s%s- %s Nexteer',NxtrConf,char(169),first,last)
      | end
  Data Store Read : DataStoreRead  DataStoreName=HwTqChAImdtCorrlnChk
  Data Store Write : DataStoreWrite  DataStoreName=HwTqChAImdtCorrlnChk
  wires:
  Data Store Read/1 -> Data Store Write/1

== system ES229A_HwTqCorrln/HwTqCorrln/HwTqCorrlnPer1/ChA  Immediate Corrleation Check /Signals Available/Imdt Corrln Chk Failed ==
  Action Port : ActionPort  ActionType=then
  Constant : Constant  Value=0  OutDataTypeStr=boolean
  CopyRight2 : Subsystem  Description=|  mask(Copyright Information){none=on}
      | Copyright info block.                                               
      |                                                                     
      | Place copyright information at the top of every subsystem in design.
      mask prompts: none "No parameters"
      mask help: Place copyright information at the top of every subsystem in design.
      mask Display:
      | NxtrConf = 'Nexteer Confidential';
      | 
      | sys = bdroot; %handle for the current model ("system")
      | first = get_param(sys,'Created');
      | first = first(end-3:end);  %year is last four digits
      | 
      | last = get_param(sys,'LastModifiedDate');
      | if isempty(last)
      |     last = datestr(now,'yyyy');
      | else
      |     last = last(end-3:end);
      | end
      | 
      | if strcmp(first,last)
      |     fprintf('%s -- Copyright %s Nexteer',NxtrConf,first)
      | else
      |     fprintf('%s -- %s%s- %s Nexteer',NxtrConf,char(169),first,last)
      | end
  Data Store Write : DataStoreWrite  DataStoreName=HwTqChAImdtCorrlnChk
  wires:
  Constant/1 -> Data Store Write/1

== system ES229A_HwTqCorrln/HwTqCorrln/HwTqCorrlnPer1/ChA  Immediate Corrleation Check /Signals Available/Imdt Corrln Chk Passed ==
  Action Port : ActionPort  ActionType=elseif
  Constant : Constant  OutDataTypeStr=boolean
  CopyRight2 : Subsystem  Description=|  mask(Copyright Information){none=on}
      | Copyright info block.                                               
      |                                                                     
      | Place copyright information at the top of every subsystem in design.
      mask prompts: none "No parameters"
      mask help: Place copyright information at the top of every subsystem in design.
      mask Display:
      | NxtrConf = 'Nexteer Confidential';
      | 
      | sys = bdroot; %handle for the current model ("system")
      | first = get_param(sys,'Created');
      | first = first(end-3:end);  %year is last four digits
      | 
      | last = get_param(sys,'LastModifiedDate');
      | if isempty(last)
      |     last = datestr(now,'yyyy');
      | else
      |     last = last(end-3:end);
      | end
      | 
      | if strcmp(first,last)
      |     fprintf('%s -- Copyright %s Nexteer',NxtrConf,first)
      | else
      |     fprintf('%s -- %s%s- %s Nexteer',NxtrConf,char(169),first,last)
      | end
  Data Store Write : DataStoreWrite  DataStoreName=HwTqChAImdtCorrlnChk
  wires:
  Constant/1 -> Data Store Write/1

== system ES229A_HwTqCorrln/HwTqCorrln/HwTqCorrlnPer1/ChA  Immediate Corrleation Check /Signals Not Available/CopyRight2 ==

== system ES229A_HwTqCorrln/HwTqCorrln/HwTqCorrlnPer1/ChB  Immediate Corrleation Check/Clear Corrln Bits/CopyRight2 ==

== system ES229A_HwTqCorrln/HwTqCorrln/HwTqCorrlnPer1/ChB  Immediate Corrleation Check/GetNtcQlfrSts/CopyRight2 ==

== system ES229A_HwTqCorrln/HwTqCorrln/HwTqCorrlnPer1/ChB  Immediate Corrleation Check/Set Corrln Bits/CopyRight2 ==

== system ES229A_HwTqCorrln/HwTqCorrln/HwTqCorrlnPer1/ChB  Immediate Corrleation Check/Signals Available/CopyRight2 ==

== system ES229A_HwTqCorrln/HwTqCorrln/HwTqCorrlnPer1/ChB  Immediate Corrleation Check/Signals Available/Hold last value ==
  Action Port : ActionPort  ActionType=else
  CopyRight2 : Subsystem  Description=|  mask(Copyright Information){none=on}
      | Copyright info block.                                               
      |                                                                     
      | Place copyright information at the top of every subsystem in design.
      mask prompts: none "No parameters"
      mask help: Place copyright information at the top of every subsystem in design.
      mask Display:
      | NxtrConf = 'Nexteer Confidential';
      | 
      | sys = bdroot; %handle for the current model ("system")
      | first = get_param(sys,'Created');
      | first = first(end-3:end);  %year is last four digits
      | 
      | last = get_param(sys,'LastModifiedDate');
      | if isempty(last)
      |     last = datestr(now,'yyyy');
      | else
      |     last = last(end-3:end);
      | end
      | 
      | if strcmp(first,last)
      |     fprintf('%s -- Copyright %s Nexteer',NxtrConf,first)
      | else
      |     fprintf('%s -- %s%s- %s Nexteer',NxtrConf,char(169),first,last)
      | end
  Data Store Read : DataStoreRead  DataStoreName=HwTqChBImdtCorrlnChk
  Data Store Write : DataStoreWrite  DataStoreName=HwTqChBImdtCorrlnChk
  wires:
  Data Store Read/1 -> Data Store Write/1

== system ES229A_HwTqCorrln/HwTqCorrln/HwTqCorrlnPer1/ChB  Immediate Corrleation Check/Signals Available/Imdt Corrln Chk Failed ==
  Action Port : ActionPort  ActionType=then
  Constant : Constant  Value=0  OutDataTypeStr=boolean
  CopyRight2 : Subsystem  Description=|  mask(Copyright Information){none=on}
      | Copyright info block.                                               
      |                                                                     
      | Place copyright information at the top of every subsystem in design.
      mask prompts: none "No parameters"
      mask help: Place copyright information at the top of every subsystem in design.
      mask Display:
      | NxtrConf = 'Nexteer Confidential';
      | 
      | sys = bdroot; %handle for the current model ("system")
      | first = get_param(sys,'Created');
      | first = first(end-3:end);  %year is last four digits
      | 
      | last = get_param(sys,'LastModifiedDate');
      | if isempty(last)
      |     last = datestr(now,'yyyy');
      | else
      |     last = last(end-3:end);
      | end
      | 
      | if strcmp(first,last)
      |     fprintf('%s -- Copyright %s Nexteer',NxtrConf,first)
      | else
      |     fprintf('%s -- %s%s- %s Nexteer',NxtrConf,char(169),first,last)
      | end
  Data Store Write : DataStoreWrite  DataStoreName=HwTqChBImdtCorrlnChk
  wires:
  Constant/1 -> Data Store Write/1

== system ES229A_HwTqCorrln/HwTqCorrln/HwTqCorrlnPer1/ChB  Immediate Corrleation Check/Signals Available/Imdt Corrln Chk Passed ==
  Action Port : ActionPort  ActionType=elseif
  Constant : Constant  OutDataTypeStr=boolean
  CopyRight2 : Subsystem  Description=|  mask(Copyright Information){none=on}
      | Copyright info block.                                               
      |                                                                     
      | Place copyright information at the top of every subsystem in design.
      mask prompts: none "No parameters"
      mask help: Place copyright information at the top of every subsystem in design.
      mask Display:
      | NxtrConf = 'Nexteer Confidential';
      | 
      | sys = bdroot; %handle for the current model ("system")
      | first = get_param(sys,'Created');
      | first = first(end-3:end);  %year is last four digits
      | 
      | last = get_param(sys,'LastModifiedDate');
      | if isempty(last)
      |     last = datestr(now,'yyyy');
      | else
      |     last = last(end-3:end);
      | end
      | 
      | if strcmp(first,last)
      |     fprintf('%s -- Copyright %s Nexteer',NxtrConf,first)
      | else
      |     fprintf('%s -- %s%s- %s Nexteer',NxtrConf,char(169),first,last)
      | end
  Data Store Write : DataStoreWrite  DataStoreName=HwTqChBImdtCorrlnChk
  wires:
  Constant/1 -> Data Store Write/1

== system ES229A_HwTqCorrln/HwTqCorrln/HwTqCorrlnPer1/ChB  Immediate Corrleation Check/Signals Not Available/CopyRight2 ==

== system ES229A_HwTqCorrln/HwTqCorrln/HwTqCorrlnPer2/ChA Long Term Correlation Fault Determination/Ch A Set//Clear Fault/Clear Fault ==
  NtcNr : Inport
  NtcStInfo : Inport  Port=2
  NtcSts : Inport  Port=3
  DebStep : Inport  Port=4
  CallDiagMgr : ActionPort  ActionType=elseif
  SetNtcSts : Subsystem  RequirementInfo={} %GIDa_fcbb9577_31d0_4d68_b123_f96b2611ba2b  TreatAsAtomicUnit=on
      settings: RTWSystemCode=Inline
  wires:
  NtcStInfo/1 -> SetNtcSts/2(NtcStInfo)
  DebStep/1 -> SetNtcSts/4(DebStep)
  NtcSts/1 -> SetNtcSts/3(NtcSts)
  NtcNr/1 -> SetNtcSts/1(NtcNr)  "NtcNr"

== system ES229A_HwTqCorrln/HwTqCorrln/HwTqCorrlnPer2/ChA Long Term Correlation Fault Determination/Ch A Set//Clear Fault/CopyRight2 ==

== system ES229A_HwTqCorrln/HwTqCorrln/HwTqCorrlnPer2/ChA Long Term Correlation Fault Determination/Ch A Set//Clear Fault/Set Fault ==
  NtcNr : Inport
  NtcStInfo : Inport  Port=2
  NtcSts : Inport  Port=3
  DebStep : Inport  Port=4
  CallDiagMgr : ActionPort  ActionType=then
  SetNtcSts : Subsystem  RequirementInfo={} %GIDa_1f2b9cd7_9f08_4317_b5c6_ae9a33518072  TreatAsAtomicUnit=on
      settings: RTWSystemCode=Inline
  wires:
  NtcNr/1 -> SetNtcSts/1(NtcNr)  "NtcNr"
  NtcSts/1 -> SetNtcSts/3(NtcSts)
  DebStep/1 -> SetNtcSts/4(DebStep)
  NtcStInfo/1 -> SetNtcSts/2(NtcStInfo)

== system ES229A_HwTqCorrln/HwTqCorrln/HwTqCorrlnPer2/ChA Long Term Correlation Fault Determination/Ch A Variable Fc Transient Fault LPF/CopyRight2 ==

== system ES229A_HwTqCorrln/HwTqCorrln/HwTqCorrlnPer2/ChA Long Term Correlation Fault Determination/ChA CMC LPF Limit/CopyRight2 ==

== system ES229A_HwTqCorrln/HwTqCorrln/HwTqCorrlnPer2/ChA Long Term Correlation Fault Determination/ChA Trq Sum Limit/CopyRight2 ==

== system ES229A_HwTqCorrln/HwTqCorrln/HwTqCorrlnPer2/ChB Long Term Correlation Fault Determination/Ch B CMC LPF Limit/CopyRight2 ==

== system ES229A_HwTqCorrln/HwTqCorrln/HwTqCorrlnPer2/ChB Long Term Correlation Fault Determination/Ch B Set//Clear Fault/Clear Fault ==
  NtcNr : Inport
  NtcStInfo : Inport  Port=2
  NtcSts : Inport  Port=3
  DebStep : Inport  Port=4
  CallDiagMgr : ActionPort  ActionType=elseif
  SetNtcSts : Subsystem  RequirementInfo={} %GIDa_5543e323_87a7_48ac_aecc_30491da2620b  TreatAsAtomicUnit=on
      settings: RTWSystemCode=Inline
  wires:
  NtcStInfo/1 -> SetNtcSts/2(NtcStInfo)
  DebStep/1 -> SetNtcSts/4(DebStep)
  NtcSts/1 -> SetNtcSts/3(NtcSts)
  NtcNr/1 -> SetNtcSts/1(NtcNr)  "NtcNr"

== system ES229A_HwTqCorrln/HwTqCorrln/HwTqCorrlnPer2/ChB Long Term Correlation Fault Determination/Ch B Set//Clear Fault/CopyRight2 ==

== system ES229A_HwTqCorrln/HwTqCorrln/HwTqCorrlnPer2/ChB Long Term Correlation Fault Determination/Ch B Set//Clear Fault/Set Fault ==
  NtcNr : Inport
  NtcStInfo : Inport  Port=2
  NtcSts : Inport  Port=3
  DebStep : Inport  Port=4
  CallDiagMgr : ActionPort  ActionType=then
  SetNtcSts : Subsystem  RequirementInfo={} %GIDa_f6d52791_8d4b_40ac_886c_26eee4cc3547  TreatAsAtomicUnit=on
      settings: RTWSystemCode=Inline
  wires:
  NtcNr/1 -> SetNtcSts/1(NtcNr)  "NtcNr"
  NtcSts/1 -> SetNtcSts/3(NtcSts)
  DebStep/1 -> SetNtcSts/4(DebStep)
  NtcStInfo/1 -> SetNtcSts/2(NtcStInfo)

== system ES229A_HwTqCorrln/HwTqCorrln/HwTqCorrlnPer2/ChB Long Term Correlation Fault Determination/Ch B Variable Fc Transient Fault LPF/CopyRight2 ==

== system ES229A_HwTqCorrln/HwTqCorrln/HwTqCorrlnPer2/ChB Long Term Correlation Fault Determination/ChB Trq Sum Limit/CopyRight2 ==

== system ES229A_HwTqCorrln/HwTqCorrln/HwTqCorrlnPer2/Independent Signals Determination/GetNtcQlfrSts/CopyRight2 ==

== system ES229A_HwTqCorrln/HwTqCorrln/HwTqCorrlnPer2/Independent Signals Determination/GetNtcQlfrSts1/CopyRight2 ==

== system ES229A_HwTqCorrln/HwTqCorrln/HwTqCorrlnPer3/ChA Long Term Offset Compensation/ChA CMC LPF/Ch A CMC LPF Hold Last Val ==
  Action Port : ActionPort  ActionType=else
  CopyRight2 : Subsystem  Description=|  mask(Copyright Information){none=on}
      | Copyright info block.                                               
      |                                                                     
      | Place copyright information at the top of every subsystem in design.
      mask prompts: none "No parameters"
      mask help: Place copyright information at the top of every subsystem in design.
      mask Display:
      | NxtrConf = 'Nexteer Confidential';
      | 
      | sys = bdroot; %handle for the current model ("system")
      | first = get_param(sys,'Created');
      | first = first(end-3:end);  %year is last four digits
      | 
      | last = get_param(sys,'LastModifiedDate');
      | if isempty(last)
      |     last = datestr(now,'yyyy');
      | else
      |     last = last(end-3:end);
      | end
      | 
      | if strcmp(first,last)
      |     fprintf('%s -- Copyright %s Nexteer',NxtrConf,first)
      | else
      |     fprintf('%s -- %s%s- %s Nexteer',NxtrConf,char(169),first,last)
      | end
  Data Store Read : DataStoreRead  DataStoreName=HwTqChACmnModCmpLpFil  DataStoreElements=HwTqChACmnModCmpLpFil.FilSt
  Out1 : Outport
  wires:
  Data Store Read/1 -> Out1/1
